simulink model "SAFracSDoF_AccResponse"  (Simulink 8.7)
settings: Solver=ode45  StartTime=0.0  StopTime=T_end  FixedStep=0.001  RelTol=1e-3
values from neighbouring files (symbols this model uses):
  dt = 0.01    [CAR_5_alpha.m]    (also in CAR_alpha.m; PGR_alpha.m; SI_d_alpha.m; SI_r_alpha.m)
  wn = 2*pi/Tn    [SI_d_alpha.m]    (also in SI_r_alpha.m; Sa_d_Tn_alpha.m = 3.14159265359; Sa_r_Tn_alpha.m = 3.14159265359)
  zeta = 0.05    [SI_d_alpha.m]    (also in SI_r_alpha.m; Sa_d_Tn_alpha.m; Sa_r_Tn_alpha.m)
undefined symbols (not defined in the file or in its folder): d, n
settings Model: Creator=ashafieezadeh3  LastModifiedBy=wang.8493  ExtModeAutoUpdateStatusClock=off
settings DataIOCC: SignalLoggingSaveFormat=ModelDataLogs
settings OptimizationCC: ExpressionDepthLimit=2147483647  InitFltsAndDblsToZero=on
settings DebuggingCC: SaveWithParameterizedLinksMsg=none  SignalResolutionControl=TryResolveAllWithWarning  SolverPrmCheckMsg=warning  MultiTaskDSMMsg=warning  MultiTaskCondExecSysMsg=none  FcnCallInpInsideContextMsg=UseLocalSettings  AllowSymbolicDim=off  StateNameClashWarn=warning
settings GRTTargetCC: TargetFcnLib=ansi_tfl_tmw.mat  GeneratePreprocessorConditionals=Use local settings  CombineOutputUpdateFcns=off  GRTInterface=on

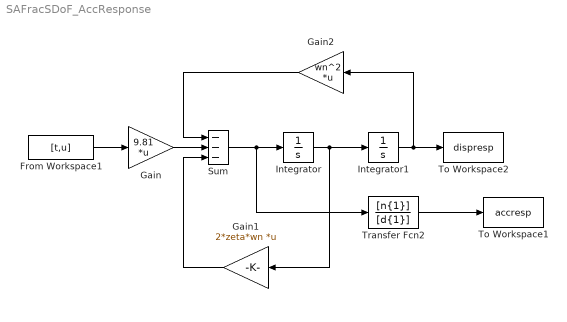
== system SAFracSDoF_AccResponse ==
  From Workspace1 : FromWorkspace  VariableName=[t,u]  SampleTime=0
  Gain : Gain  Gain=9.81  Multiplication=Matrix(K*u)
  Gain1 : Gain  Gain=2*zeta*wn  Multiplication=Matrix(K*u)
  Gain2 : Gain  Gain=wn^2  Multiplication=Matrix(K*u)
  Integrator : Integrator
  Integrator1 : Integrator
  Sum : Sum  Inputs=---
  To Workspace1 : ToWorkspace  VariableName=accresp  SampleTime=dt
  To Workspace2 : ToWorkspace  VariableName=dispresp  SampleTime=dt
  Transfer Fcn2 : TransferFcn  Numerator=[n{1}]  Denominator=[d{1}]
  wires:
  From Workspace1/1 -> Gain/1
  Integrator1/1 -> To Workspace2/1, Gain2/1
  Gain/1 -> Sum/2
  Integrator/1 -> Integrator1/1, Gain1/1
  Sum/1 -> Transfer Fcn2/1, Integrator/1
  Gain1/1 -> Sum/3
  Gain2/1 -> Sum/1
  Transfer Fcn2/1 -> To Workspace1/1
